simulink model "simulink_models_for_lab_4"  (R2024b)
settings: Solver=VariableStepAuto  StartTime=0.0  StopTime=7.0  RelTol=1e-3
libraries: simulink x5
settings Model: Creator=cloud  LastModifiedBy=cloud

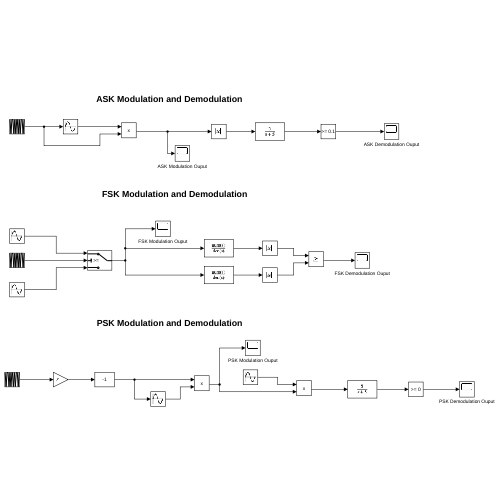
[thumbnail: Simulink's stored preview of the top-level diagram]
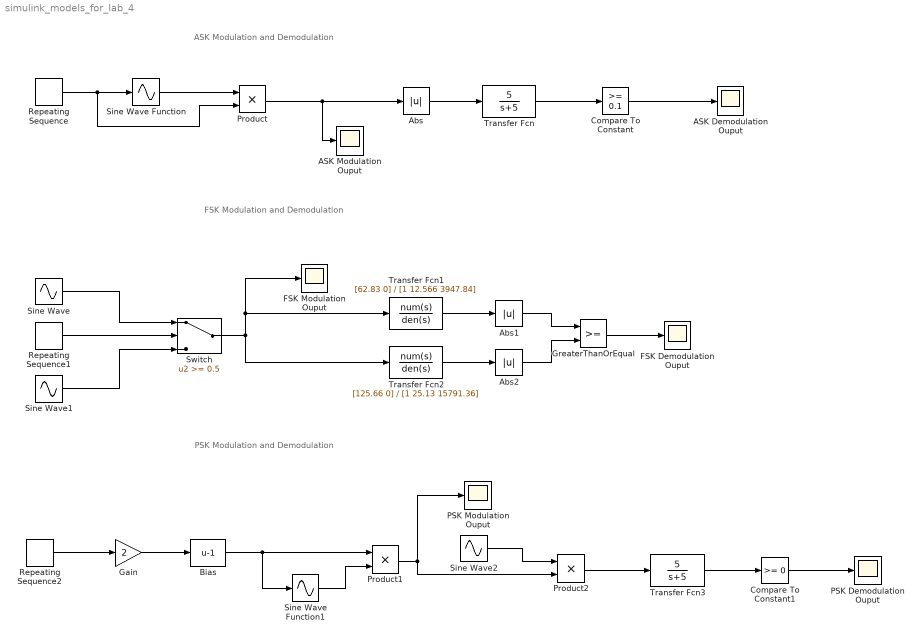
== system simulink_models_for_lab_4 ==
  note: FSK Modulation and Demodulation
  note: ASK Modulation and Demodulation
  note: PSK Modulation and Demodulation
  ASK Demodulation Ouput : Scope
  ASK Modulation Ouput : Scope
  Abs : Abs  SaturateOnIntegerOverflow=off
  Abs1 : Abs  SaturateOnIntegerOverflow=off
  Abs2 : Abs  SaturateOnIntegerOverflow=off
  Bias : Bias  Bias=-1  SaturateOnIntegerOverflow=off
  Compare To Constant : simulink/Logic and Bit Operations/Compare To Constant  relop=>=  const=0.1  OutDataTypeStr=boolean
  Compare To Constant1 : simulink/Logic and Bit Operations/Compare To Constant  relop=>=  const=0  OutDataTypeStr=boolean
  FSK Demodulation Ouput : Scope
  FSK Modulation Ouput : Scope
  Gain : Gain  Gain=2
  GreaterThanOrEqual : RelationalOperator  OutDataTypeStr=boolean  RndMeth=Simplest  InputSameDT=off
  PSK Demodulation Ouput : Scope
  PSK Modulation Ouput : Scope
  Product : Product
  Product1 : Product
  Product2 : Product
  Repeating Sequence : simulink/Sources/Repeating Sequence  rep_seq_t=[0 1 2 3 4 5]  rep_seq_y=[1 0 1 1 0 1]
  Repeating Sequence1 : simulink/Sources/Repeating Sequence  rep_seq_t=[0 1 2 3 4 5]  rep_seq_y=[1 0 1 1 0 1]
  Repeating Sequence2 : simulink/Sources/Repeating Sequence  rep_seq_t=[0 1 2 3 4 5]  rep_seq_y=[1 0 1 1 0 1]
  Sine Wave : Sin  Frequency=20  SampleTime=0
  Sine Wave Function : Sin  TimeSource=Use external signal  Frequency=10  SampleTime=0
  Sine Wave Function1 : Sin  TimeSource=Use external signal  Frequency=10  SampleTime=0
  Sine Wave1 : Sin  Frequency=10  SampleTime=0
  Sine Wave2 : Sin  Frequency=10  SampleTime=0
  Switch : Switch  Threshold=0.5  SaturateOnIntegerOverflow=off  InputSameDT=off
  Transfer Fcn : TransferFcn  Numerator=[5]  Denominator=[1 5]
  Transfer Fcn1 : TransferFcn  Numerator=[62.83 0]  Denominator=[1 12.566 3947.84]
  Transfer Fcn2 : TransferFcn  Numerator=[125.66 0]  Denominator=[1 25.13 15791.36]
  Transfer Fcn3 : TransferFcn  Numerator=[5]  Denominator=[1 5]
  wires:
  Repeating Sequence/1 -> Product/2, Sine Wave Function/1
  Sine Wave Function/1 -> Product/1
  Product/1 -> ASK Modulation Ouput/1, Abs/1
  Abs/1 -> Transfer Fcn/1
  Transfer Fcn/1 -> Compare To Constant/1
  Compare To Constant/1 -> ASK Demodulation Ouput/1
  Sine Wave/1 -> Switch/1
  Repeating Sequence1/1 -> Switch/2
  Sine Wave1/1 -> Switch/3
  Switch/1 -> FSK Modulation Ouput/1, Transfer Fcn1/1, Transfer Fcn2/1
  Transfer Fcn2/1 -> Abs2/1
  Transfer Fcn1/1 -> Abs1/1
  Abs1/1 -> GreaterThanOrEqual/1
  Abs2/1 -> GreaterThanOrEqual/2
  GreaterThanOrEqual/1 -> FSK Demodulation Ouput/1
  Repeating Sequence2/1 -> Gain/1
  Gain/1 -> Bias/1
  Bias/1 -> Sine Wave Function1/1, Product1/1
  Sine Wave Function1/1 -> Product1/2
  Product1/1 -> Product2/2, PSK Modulation Ouput/1
  Sine Wave2/1 -> Product2/1
  Product2/1 -> Transfer Fcn3/1
  Transfer Fcn3/1 -> Compare To Constant1/1
  Compare To Constant1/1 -> PSK Demodulation Ouput/1
